simulink model "datalogger_host"  (R2021a)
settings: Solver=FixedStepDiscrete  StartTime=0.0  StopTime=inf  RelTol=1e-3  EnableMultiTasking=on
libraries: instrumentseriallib x3
settings Model: Creator=61301765  LastModifiedBy=61301765
settings OptimizationCC: DefaultParameterBehavior=Inlined  DefaultUnderspecifiedDataType=single  EnhancedBackFolding=on  PassReuseOutputArgsAs=Individual arguments  ZeroExternalMemoryAtStartup=off  MaxStackSize=64  OptimizeBlockOrder=speed  DifferentSizesBufferReuse=on  OptimizationCustomize=off  EfficientTunableParamExpr=on
settings DebuggingCC: ParameterTunabilityLossMsg=error
settings HardwareCC: ProdBitPerChar=16  ProdBitPerInt=16  ProdBitPerPointer=32  ProdBitPerSizeT=32  ProdBitPerPtrDiffT=32  ProdLargestAtomicInteger=Integer  ProdLargestAtomicFloat=None  ProdWordSize=16  ProdLongLongMode=on  ProdHWDeviceType=Texas Instruments->C2000
settings SFSimCC: MATLABDynamicMemAlloc=off
settings RTWCC: SystemTargetFile=ert.tlc  TemplateMakefile=ert_default_tmf  Toolchain=Texas Instruments Code Composer Studio (C2000)
settings CodeAppCC: ForceParamTrailComments=on  IgnoreCustomStorageClasses=off  OperatorAnnotations=on  SimulinkDataObjDesc=on  SFDataObjDesc=on  InsertBlockDesc=on
settings ERTTargetCC: ExtModeStaticAllocSize=5000  ERTCustomFileTemplate=example_file_process.tlc

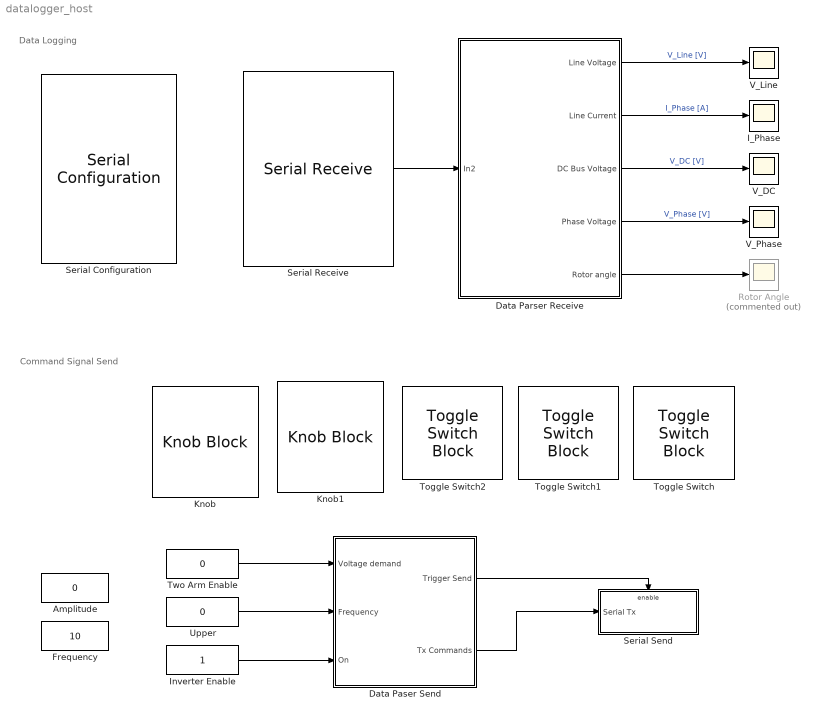
== system datalogger_host ==
  note: Data Logging
  note: Command Signal Send
  Amplitude : Constant  Value=0  VectorParams1D=off  OutDataTypeStr=single  SampleTime=0.06
  Data Parser Receive : Subsystem
  Data Paser Send : Subsystem
  Frequency : Constant  Value=10  VectorParams1D=off  OutDataTypeStr=single  SampleTime=0.06
  I_Phase : Scope
  Inverter Enable : Constant  VectorParams1D=off  OutDataTypeStr=single  SampleTime=0.06
  Knob : KnobBlock  ScaleMax=6
  Knob1 : KnobBlock  ScaleMin=-100
  Rotor Angle : Scope  Commented=on
  Serial Configuration : instrumentseriallib/Serial Configuration  Priority=-200000  Port=COM6  ComPort=COM6  BaudRate=6250000  DataBits=8  Parity=none  StopBits=1  ByteOrder=little-endian  FlowControl=none  Timeout=1  SimulateUsing=Interpreted execution  BlockInModel=on
  Serial Receive : instrumentseriallib/Serial Receive  Port=COM6  ComPort=COM6  DataType=uint16  SaveDataType=uint8  ToggleHeader=on  Header=[1 1]  ToggleTerminator=on  Terminator=Custom terminator  CustomTerminator=[2 2]  ToggleDataSize=on  DataSize="[1  12000*7]"  EnableBlockingMode=on  ActionDataUnavailable=Output last received value  ActionWhenDataUnavailable=Output last received value  CustomValue=0  SampleTime=0.06  SimulateUsing=Interpreted execution  BlockInModel=on
  Serial Send : Subsystem  TreatAsAtomicUnit=on
  Toggle Switch : ToggleSwitchBlock
      settings: Values={{'Off', 'On'}, [0 1]}
  Toggle Switch1 : ToggleSwitchBlock
      settings: Values={{'Off', 'On'}, [0 1]}
  Toggle Switch2 : ToggleSwitchBlock
      settings: Values={{'Off', 'On'}, [0 1]}
  Two Arm Enable : Constant  Value=0  VectorParams1D=off  OutDataTypeStr=single  SampleTime=0.06
  Upper : Constant  Value=0  VectorParams1D=off  OutDataTypeStr=single  SampleTime=0.06
  V_DC : Scope
  V_Line : Scope
  V_Phase : Scope
  wires:
  Serial Receive/1 -> Data Parser Receive/1(In2)
  Data Parser Receive/1(Line Voltage) -> V_Line/1  "V_Line [V]"
  Data Parser Receive/2(Line Current) -> I_Phase/1  "I_Phase [A]"
  Data Parser Receive/3(DC Bus Voltage) -> V_DC/1  "V_DC [V]"
  Data Paser Send/2(Tx Commands) -> Serial Send/1(Serial Tx)
  Data Paser Send/1(Trigger Send) -> Serial Send/Enable
  Inverter Enable/1 -> Data Paser Send/3(On)
  Data Parser Receive/4(Phase Voltage) -> V_Phase/1  "V_Phase [V]"
  Data Parser Receive/5(Rotor angle) -> Rotor Angle/1
  Two Arm Enable/1 -> Data Paser Send/1(Voltage demand)
  Upper/1 -> Data Paser Send/2(Frequency)

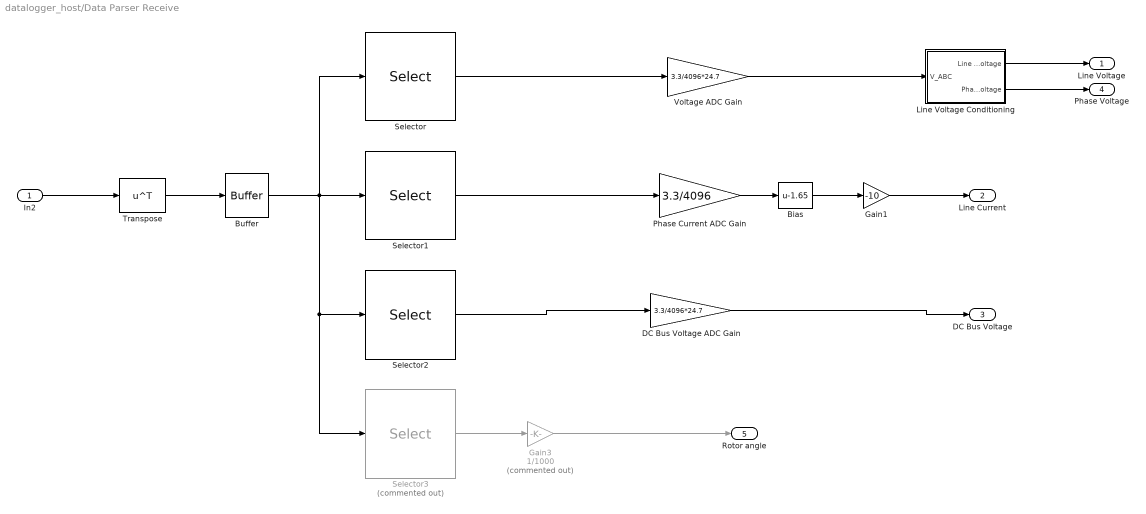
== system datalogger_host/Data Parser Receive ==
  In2 : Inport
  Bias : Bias  Bias=-1.65
  Buffer : Buffer  N=7  OutputFrames=off
  DC Bus Voltage ADC Gain : Gain  Gain=3.3/4096*24.7  ParamMin=[0]  ParamMax=[81.51]  OutDataTypeStr=single
  Gain1 : Gain  Gain=-10
  Gain3 : Gain  Commented=on  Gain=1/1000
  Line Voltage Conditioning : Subsystem
  Phase Current ADC Gain : Gain  Gain=3.3/4096  ParamMin=[0]  ParamMax=[3.3]  OutDataTypeStr=single
  Selector : Selector  InputPortWidth=7  IndexOptions=Index vector (dialog)  Indices=[1 2 3]  OutputSizes=1
  Selector1 : Selector  InputPortWidth=7  IndexOptions=Index vector (dialog)  Indices=[4 5 6]  OutputSizes=1
  Selector2 : Selector  InputPortWidth=7  IndexOptions=Index vector (dialog)  Indices=7  OutputSizes=1
  Selector3 : Selector  Commented=on  InputPortWidth=11  IndexOptions=Index vector (dialog)  Indices=[8 9 10]  OutputSizes=1
  Transpose : Math  Operator=transpose  SignedPower=on  SaturateOnIntegerOverflow=on
  Voltage ADC Gain : Gain  Gain=3.3/4096*24.7  ParamMin=[0]  ParamMax=[81.51]  OutDataTypeStr=single
  Line Voltage : Outport  VectorParamsAs1DForOutWhenUnconnected=off
  Line Current : Outport  Port=2  VectorParamsAs1DForOutWhenUnconnected=off
  DC Bus Voltage : Outport  Port=3  VectorParamsAs1DForOutWhenUnconnected=off
  Phase Voltage : Outport  Port=4
  Rotor angle : Outport  Port=5
  wires:
  In2/1 -> Transpose/1
  Transpose/1 -> Buffer/1
  Buffer/1 -> Selector2/1, Selector3/1, Selector1/1, Selector/1
  Line Voltage Conditioning/1(Line Voltage) -> Line Voltage/1
  Line Voltage Conditioning/2(Phase Voltage) -> Phase Voltage/1
  Selector3/1 -> Gain3/1
  Gain3/1 -> Rotor angle/1
  Selector1/1 -> Phase Current ADC Gain/1
  Bias/1 -> Gain1/1
  DC Bus Voltage ADC Gain/1 -> DC Bus Voltage/1
  Gain1/1 -> Line Current/1
  Phase Current ADC Gain/1 -> Bias/1
  Selector2/1 -> DC Bus Voltage ADC Gain/1
  Selector/1 -> Voltage ADC Gain/1
  Voltage ADC Gain/1 -> Line Voltage Conditioning/1(V_ABC)

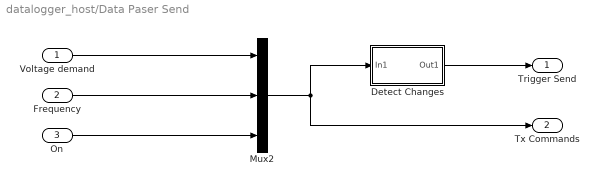
== system datalogger_host/Data Paser Send ==
  Voltage demand : Inport
  Frequency : Inport  Port=2
  On : Inport  Port=3
  Detect Changes : Subsystem
  Mux2 : Mux  Inputs=3
  Trigger Send : Outport  VectorParamsAs1DForOutWhenUnconnected=off
  Tx Commands : Outport  Port=2  VectorParamsAs1DForOutWhenUnconnected=off
  wires:
  Mux2/1 -> Tx Commands/1, Detect Changes/1(In1)
  Detect Changes/1(Out1) -> Trigger Send/1
  On/1 -> Mux2/3
  Voltage demand/1 -> Mux2/1
  Frequency/1 -> Mux2/2

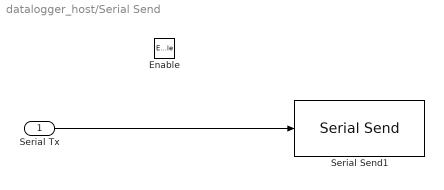
== system datalogger_host/Serial Send ==
  Serial Tx : Inport
  Enable : EnablePort
  Serial Send1 : instrumentseriallib/Serial Send  Port=COM6  ComPort=COM6  Header=[ 83 ]  Terminator=Custom terminator  CustomTerminator=[ 69 ]  EnableBlockingMode=on  SimulateUsing=Interpreted execution  BlockInModel=on
  wires:
  Serial Tx/1 -> Serial Send1/1

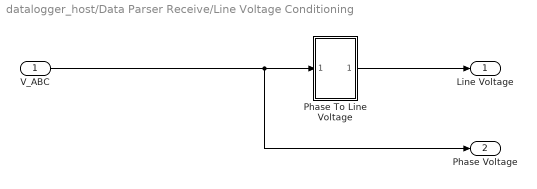
== system datalogger_host/Data Parser Receive/Line Voltage Conditioning ==
  V_ABC : Inport
  Phase To Line Voltage : Subsystem
  Line Voltage : Outport
  Phase Voltage : Outport  Port=2
  wires:
  V_ABC/1 -> Phase Voltage/1, Phase To Line Voltage/1(In1)
  Phase To Line Voltage/1(Out1) -> Line Voltage/1

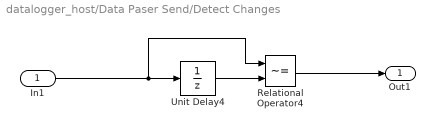
== system datalogger_host/Data Paser Send/Detect Changes ==
  In1 : Inport
  Relational Operator4 : RelationalOperator  Operator=~=  OutDataTypeStr=boolean  RndMeth=Nearest
  Unit Delay4 : UnitDelay  SampleTime=-1  HasFrameUpgradeWarning=on
  Out1 : Outport  VectorParamsAs1DForOutWhenUnconnected=off
  wires:
  Unit Delay4/1 -> Relational Operator4/2
  In1/1 -> Relational Operator4/1, Unit Delay4/1
  Relational Operator4/1 -> Out1/1

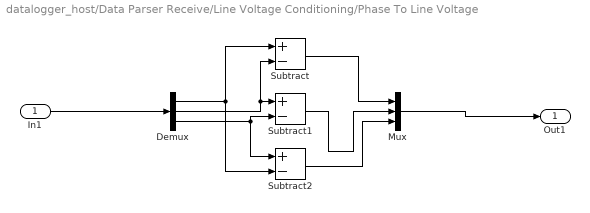
== system datalogger_host/Data Parser Receive/Line Voltage Conditioning/Phase To Line Voltage ==
  In1 : Inport
  Demux : Demux  Outputs=3
  Mux : Mux  Inputs=3
  Subtract : Sum  Inputs=+-
  Subtract1 : Sum  Inputs=+-
  Subtract2 : Sum  Inputs=+-
  Out1 : Outport
  wires:
  Demux/1 -> Subtract2/2, Subtract/1
  In1/1 -> Demux/1
  Subtract/1 -> Mux/1
  Mux/1 -> Out1/1
  Demux/2 -> Subtract/2, Subtract1/1
  Subtract1/1 -> Mux/2
  Subtract2/1 -> Mux/3
  Demux/3 -> Subtract1/2, Subtract2/1
